simulink model "Kalman_FullSystem"  (R2024a)
settings: Solver=FixedStepAuto  StartTime=0.0  StopTime=0.05  FixedStep=0.05  RelTol=1e-3
model workspace (MAT data in the model file):
  Delta_t = 0.1
  J1 = 0.833333333333
  J2 = 1.08333333333
  J3 = 0.416666666667
  NoiseCov = [0.5  0  0  0  0  0; 0  0.5  0  0  0  0; 0  0  0.5  0  0  0; 0  0  0  0.5  0  0; 0  0  0  0  0.5  0; 0  0  0  0  0  0.5]
  Orbit_Incl = 51.6
  Q_identity = [0.05  0  0  0  0  0  0; 0  0.05  0  0  0  0  0; 0  0  0.05  0  0  0  0; 0  0  0  0.05  0  0  0; 0  0  0  0  0.05  0  0; 0  0  0  0  0  0.05  0; 0  0  0  0  0  0  0.05]
  Sig = Simulink.Signal
  Sig.DataType = 'auto'
  Sig.Dimensions = -1
  Sig.DimensionsMode = 'auto'
  Sig.Complexity = 'auto'
  Sig.SampleTime = -1
  Sig.SamplingMode = 'auto'
  Sig1 = Simulink.Signal
  Sig1.DataType = 'auto'
  Sig1.Dimensions = -1
  Sig1.DimensionsMode = 'auto'
  Sig1.Complexity = 'auto'
  Sig1.SampleTime = -1
  Sig1.SamplingMode = 'auto'
  controlRun = 1
  jd_input = 2458850.00006
  m = 100
  n = 7
  prev_torque_input = [4.02125178476e-05; -0.000240074266532; 0.000969921285444]
  q_ff_in = [0.768162333731 -0.000607721012165 0.00073835510125 -0.64025441392]
  q_mea = [0.201779427007 -0.600440780835 -0.499157225709 -0.59126812494]
  s_input = [0.0589841167561  0.00581351479597  0.00668594935891  -0.00630732370495  0.000663483023899  0.00184880164458  0.000570366934632; 0.00581351479597  0.0937594050574  0.0387635496011  -0.0430050360951  0.000555134956355  0.00180643488778  -0.00190339065861; 0.00668594935891  0.0387635496011  0.103662181174  -0.0426676946457  -0.0011343563344  0.00228890389951  0.000237159003537; -0.00630732370495  -0.0430050360951  -0.0426676946457  0.116378630936  0.0019375862402  -0.00189390453411  0.00103186473468; 0.000663483023899  0.000555134956355  -0.0011343563344  0.0019375862402  0.134971771072  -0.000682723438692  0.000145669100888; 0.00184880164458  0.00180643488778  0.00228890389951  -0.00189390453411  -0.000682723438692  0.134976824741  -0.00135891657435; 0.000570366934632  -0.00190339065861  0.000237159003537  0.00103186473468  0.000145669100888  -0.00135891657435  0.134973743075]
  s_input_cons = [1.94870414  1.25588909  1.4416761  1.0780205  1.49168854  1.53894753  1.37981514; 1.25588909  2.30599344  1.57766712  1.62980068  1.46050557  1.31460547  1.13813509; 1.4416761  1.57766712  1.70958392  1.12140846  1.38322267  1.58836736  1.34392315; 1.0780205  1.62980068  1.12140846  1.77837393  1.21690337  0.94427956  1.46043147; 1.49168854  1.46050557  1.38322267  1.21690337  2.06327445  1.39185931  1.33424815; 1.53894753  1.31460547  1.58836736  0.94427956  1.39185931  2.02772691  1.7277207; 1.37981514  1.13813509  1.34392315  1.46043147  1.33424815  1.7277207  2.16380015]
  savedTorque = [0.000657725470141; -0.000240297847613; -0.000713900658607]
  t_step = 0.05
  v_icrf_input = [-949481.777156 -889776.036157 4371.77407199]
  w_mea = [0.000477892534013 0.0173144207751 0.0745768968359]
  x_icrf_input = [-3388291.56974 3592736.49121 -4663347.3899]
  x_icrf_input_cons = [3649700 3308200 -4676600]
  x_input = [0.411501608148; -0.308732372219; -0.291057996427; -0.806620103613; -0.492262126493; 0.179846356615; 0.534305378558]
  x_input_cons = [0.2; 0.6; 0.5; 0.59160797831; 0.1; 0.4; 0.9]
libraries: aerolibsatdyn x2, aerolibtransform2 x2, aerolibutil x2
settings Model: Creator=alenachan  LastModifiedBy=ruimi

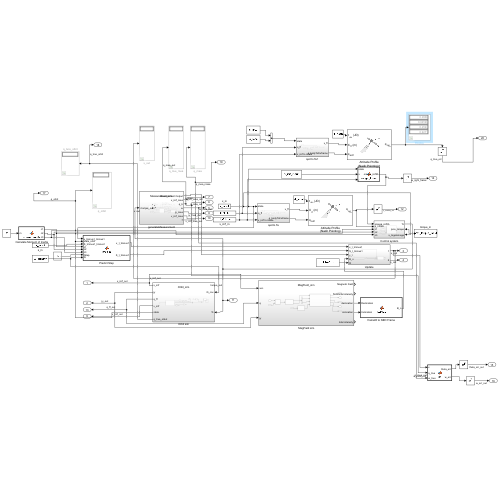
[thumbnail: Simulink's stored preview of the top-level diagram]
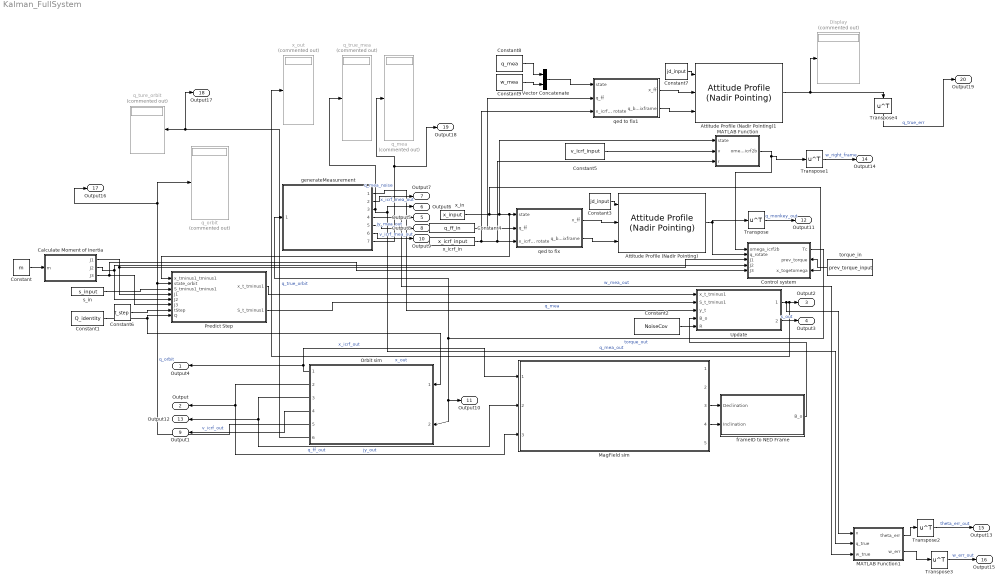
== system Kalman_FullSystem ==
  " Calculate Moment of Inertia" : MATLAB Function  Priority=10  TreatAsAtomicUnit=on
  Attitude Profile (Nadir Pointing) : aerolibsatdyn/Attitude Profile (Nadir Pointing)  Priority=3  outputError=on  outputFinalAttitude=off  portFrame=Fixed-frame  pointingMode=Custom  celestialTarget=Sun  tunablePointing=off  primaryAlignmentSrc=Dialog  primaryAlignment=[0 0 1]  secondaryAlignmentSrc=Dialog  secondaryAlignment=[1 0 0]  constraintFrame=ICRF  primaryConstraintSrc=Dialog  primaryConstraint=[1 0 0]  secondaryConstraintSrc=Dialog  secondaryConstraint=[0 1 0]
  Attitude Profile (Nadir Pointing)1 : aerolibsatdyn/Attitude Profile (Nadir Pointing)  Priority=3  outputError=on  outputFinalAttitude=off  portFrame=Fixed-frame  pointingMode=Custom  celestialTarget=Sun  tunablePointing=off  primaryAlignmentSrc=Dialog  primaryAlignment=[0 0 1]  secondaryAlignmentSrc=Dialog  secondaryAlignment=[1 0 0]  constraintFrame=ICRF  primaryConstraintSrc=Dialog  primaryConstraint=[1 0 0]  secondaryConstraintSrc=Dialog  secondaryConstraint=[0 1 0]
  Constant : Constant  Value=m
  Constant1 : Constant  Value=Q_identity
  Constant2 : Constant  Value=NoiseCov
  Constant3 : Constant  Value=jd_input
  Constant4 : Constant  Value=q_ff_in
  Constant5 : Constant  Value=v_icrf_input
  Constant6 : Constant  Value=t_step
  Constant7 : Constant  Value=jd_input
  Constant8 : Constant  Value=q_mea
  Constant9 : Constant  Value=w_mea
  Control system : Subsystem  Priority=4
      settings: PortSchema="{\"entries\":[{\"content\":{\"sides\":[{\"content\":{\"connectorIds\":[\"In1\",\"In2\",\"In3\",\"In4\",\"In5\"]},\"type\":\"ConnectorPlacement.EquallySpacedRectSide\",\"uuid\":\"8eb5f269-cc65-4267-936a-9f0f4ccd4d18\"},{\"content\":{\"connectorIds\":[\"Out1\",\"In6\",\"In7\"],\"side\":\"RIGHT\"},\"type\":\"ConnectorPlacement.EquallySpacedRectSide\",\"uuid\":\"3df96c14-e4ae-45ba-8fc0-de3a9fdcf55a\"},{\"content\":{\"side\":\"TOP\"},\"type\":\"ConnectorPlacement.EquallySpacedRectSide\",\"uuid\":\"e3effbcc-2fcc-4dea-811c-5aa639521533\"}]},\"type\":\"ConnectorPlacement.EquallySpacedConnector\",\"uuid\":\"93bbc224-b85a-4291-8bf8-2645c40efc9b\"}],\"packageUris\":[\"http://schema.mathworks.com/mf0/Connector/R2020b\"],\"version\":\"1.0\"}"
  Display : Display  Commented=on
  MATLAB Function : MATLAB Function  TreatAsAtomicUnit=on
  MATLAB Function1 : MATLAB Function  TreatAsAtomicUnit=on
  MagField sim : Subsystem  Priority=8  ReferencedSubsystem=MagField_sim
  Orbit sim : Subsystem  Priority=7  ReferencedSubsystem=Orbit_sim
  Predict Step : MATLAB Function  Priority=11  TreatAsAtomicUnit=on
  Transpose{,1..4} (5 alike) : Math  Operator=transpose
  Update : Subsystem  Priority=12
  Vector Concatenate : Concatenate
  frameID to NED Frame : MATLAB Function  Priority=9  TreatAsAtomicUnit=on
  generateMeasurement : Subsystem  Priority=5  ReferencedSubsystem=Measurement_sim
  q_mea : Display  Commented=on
  q_orbit : Display  Commented=on
  q_true_mea : Display  Commented=on
  q_ture_orbit : Display  Commented=on
  qed to fix : Subsystem  Priority=2
  qed to fix1 : Subsystem  Priority=2
  s_in : Constant  Priority=1  Value=s_input
  torque_in : Constant  Value=prev_torque_input
  x_icrf_in : Constant  Value=x_icrf_input
  x_in : Constant  Value=x_input
  x_out : Display  Commented=on
  Output4 : Outport
  Output : Outport  Port=2
  Output2 : Outport  Port=3
  Output3 : Outport  Port=4
  Output5 : Outport  Port=5
  Output6 : Outport  Port=6
  Output7 : Outport  Port=7
  Output8 : Outport  Port=8
  Output1 : Outport  Port=9
  Output9 : Outport  Port=10
  Output10 : Outport  Port=11
  Output11 : Outport  Port=12
  Output12 : Outport  Port=13
  Output14 : Outport  Port=14
  Output13 : Outport  Port=15
  Output15 : Outport  Port=16
  Output16 : Outport  Port=17
  Output17 : Outport  Port=18
  Output18 : Outport  Port=19
  Output19 : Outport  Port=20
  wires:
  Control system/1(Tc) -> Output10/1, Orbit sim/2, generateMeasurement/1  "torque_out"
  MagField sim/3 -> frameID to NED Frame/1(Declination)
  MagField sim/4 -> frameID to NED Frame/2(Inclination)
  frameID to NED Frame/1(B_o) -> Update/4(B_o)
  Orbit sim/2 -> MagField sim/3, Output/1  "jy_out"
  Orbit sim/1 -> MagField sim/1, Output4/1  "x_icrf_out"
  Constant/1 -> " Calculate Moment of Inertia"/1(m)
  " Calculate Moment of Inertia"/1(J1) -> Predict Step/4(J1), Control system/3(J1)
  " Calculate Moment of Inertia"/2(J2) -> Control system/4(J2), Predict Step/5(J2)
  " Calculate Moment of Inertia"/3(J3) -> Predict Step/6(J3), Control system/5(J3)
  Constant1/1 -> Orbit sim/1, Predict Step/8(Q)
  x_in/1 -> Control system/7(x_togetomega), MATLAB Function/1(state), Predict Step/1(x_tminus1_tminus1), qed to fix/1(state)
  s_in/1 -> Predict Step/3(S_tminus1_tminus1)
  x_icrf_in/1 -> qed to fix1/3(x_icrf to rotate), MATLAB Function/3(r), qed to fix/3(x_icrf to rotate)
  Predict Step/1(x_t_tminus1) -> Update/1(x_t_tminus1)
  Predict Step/2(S_t_tminus1) -> Update/2(S_t_tminus1)
  Constant2/1 -> Update/5(R)
  Update/1(1) -> MATLAB Function1/1(x), x_out/1, Output2/1  "x_out"
  Update/2(2) -> Output3/1  "s_out"
  Orbit sim/3 -> MagField sim/2, Output12/1  "q_ff_out"
  generateMeasurement/2 -> Output7/1  "x_icrf_mea_out"
  generateMeasurement/5 -> Output8/1  "jy_mea_out"
  Orbit sim/4 -> Output1/1  "v_icrf_out"
  generateMeasurement/6 -> Output9/1  "v_icrf_mea_out"
  torque_in/1 -> Control system/6(prev_torque)
  Transpose/1 -> Output11/1  "q_monkey_out"
  Constant3/1 -> Attitude Profile (Nadir Pointing)/1
  qed to fix/2(q_bodyToFixframe) -> Attitude Profile (Nadir Pointing)/3
  Constant4/1 -> qed to fix1/2(q_ff), qed to fix/2(q_ff)
  qed to fix/1(x_ff) -> Attitude Profile (Nadir Pointing)/2
  Constant6/1 -> Predict Step/7(tStep)
  Orbit sim/5 -> Output16/1, q_orbit/1, Predict Step/2(state_orbit)  "q_orbit"
  Attitude Profile (Nadir Pointing)/1 -> Transpose/1, Control system/2(q_rotate)
  Constant5/1 -> MATLAB Function/2(v)
  MATLAB Function/1(omega_icrf2b) -> Transpose1/1, Control system/1(omega_icrf2b)
  Transpose1/1 -> Output14/1  "w_right_frame"
  Transpose2/1 -> Output13/1  "theta_err_out"
  MATLAB Function1/2(w_err) -> Transpose3/1
  Transpose3/1 -> Output15/1  "w_err_out"
  generateMeasurement/4 -> MATLAB Function1/3(w_true), Output5/1  "w_mea_out"
  generateMeasurement/3 -> Output6/1, MATLAB Function1/2(q_true), q_true_mea/1  "q_mea_out"
  MATLAB Function1/1(theta_err) -> Transpose2/1
  Orbit sim/6 -> Output17/1, q_ture_orbit/1  "q_true_orbit"
  generateMeasurement/1 -> Update/3(y_t)  "q_mea"
  generateMeasurement/7 -> Output18/1, q_mea/1  "q_mea_noise"
  Constant7/1 -> Attitude Profile (Nadir Pointing)1/1
  qed to fix1/1(x_ff) -> Attitude Profile (Nadir Pointing)1/2
  qed to fix1/2(q_bodyToFixframe) -> Attitude Profile (Nadir Pointing)1/3
  Constant8/1 -> Vector Concatenate/1
  Constant9/1 -> Vector Concatenate/2
  Vector Concatenate/1 -> qed to fix1/1(state)
  Attitude Profile (Nadir Pointing)1/1 -> Display/1, Transpose4/1
  Transpose4/1 -> Output19/1  "q_true_err"

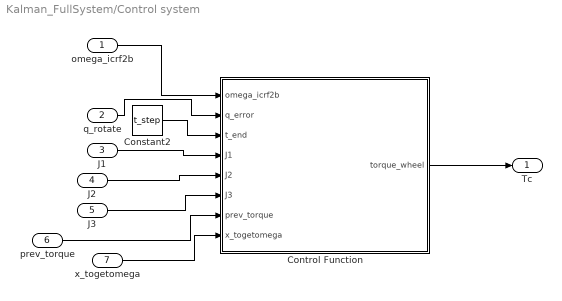
== system Kalman_FullSystem/Control system ==
  omega_icrf2b : Inport
  q_rotate : Inport  Port=2
  J1 : Inport  Port=3
  J2 : Inport  Port=4
  J3 : Inport  Port=5
  prev_torque : Inport  Port=6
  x_togetomega : Inport  Port=7
  Constant2 : Constant  Value=t_step
  Control Function : MATLAB Function  TreatAsAtomicUnit=on
  Tc : Outport
  wires:
  Constant2/1 -> Control Function/3(t_end)
  Control Function/1(torque_wheel) -> Tc/1
  q_rotate/1 -> Control Function/2(q_error)
  J1/1 -> Control Function/4(J1)
  J2/1 -> Control Function/5(J2)
  J3/1 -> Control Function/6(J3)
  prev_torque/1 -> Control Function/7(prev_torque)
  x_togetomega/1 -> Control Function/8(x_togetomega)
  omega_icrf2b/1 -> Control Function/1(omega_icrf2b)

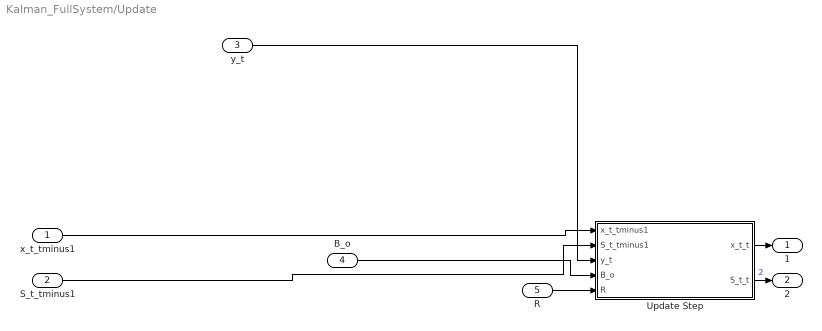
== system Kalman_FullSystem/Update ==
  x_t_tminus1 : Inport
  S_t_tminus1 : Inport  Port=2
  y_t : Inport  Port=3
  B_o : Inport  Port=4
  R : Inport  Port=5
  Update Step : MATLAB Function  TreatAsAtomicUnit=on
  1 : Outport
  2 : Outport  Port=2
  wires:
  y_t/1 -> Update Step/3(y_t)
  Update Step/2(S_t_t) -> 2/1  "2"
  B_o/1 -> Update Step/4(B_o)
  S_t_tminus1/1 -> Update Step/2(S_t_tminus1)
  x_t_tminus1/1 -> Update Step/1(x_t_tminus1)
  R/1 -> Update Step/5(R)
  Update Step/1(x_t_t) -> 1/1

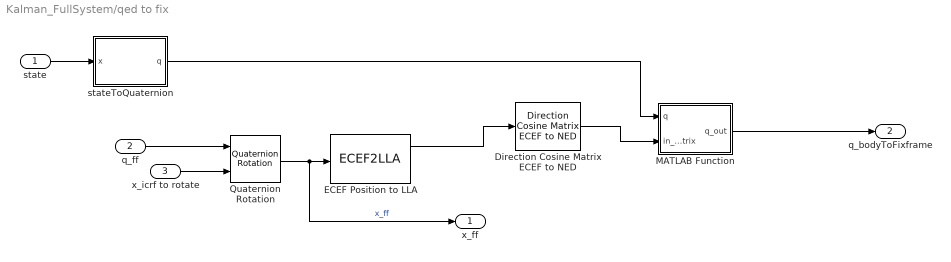
== system Kalman_FullSystem/qed to fix ==
  state : Inport
  q_ff : Inport  Port=2
  x_icrf to rotate : Inport  Port=3
  Direction Cosine Matrix ECEF to NED : aerolibtransform2/Direction Cosine Matrix ECEF to NED
  ECEF Position to LLA : ECEF2LLA
  MATLAB Function : MATLAB Function  TreatAsAtomicUnit=on
  Quaternion Rotation : aerolibutil/Quaternion Rotation
  stateToQuaternion : MATLAB Function  TreatAsAtomicUnit=on
  x_ff : Outport
  q_bodyToFixframe : Outport  Port=2
  wires:
  state/1 -> stateToQuaternion/1(x)
  Quaternion Rotation/1 -> x_ff/1, ECEF Position to LLA/1  "x_ff"
  x_icrf to rotate/1 -> Quaternion Rotation/2
  ECEF Position to LLA/1 -> Direction Cosine Matrix ECEF to NED/1
  Direction Cosine Matrix ECEF to NED/1 -> MATLAB Function/2(in_matrix)
  stateToQuaternion/1(q) -> MATLAB Function/1(q)
  MATLAB Function/1(q_out) -> q_bodyToFixframe/1
  q_ff/1 -> Quaternion Rotation/1

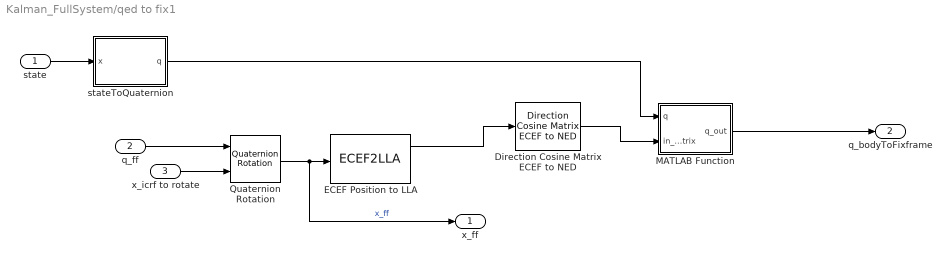
== system Kalman_FullSystem/qed to fix1 ==
  state : Inport
  q_ff : Inport  Port=2
  x_icrf to rotate : Inport  Port=3
  Direction Cosine Matrix ECEF to NED : aerolibtransform2/Direction Cosine Matrix ECEF to NED
  ECEF Position to LLA : ECEF2LLA
  MATLAB Function : MATLAB Function  TreatAsAtomicUnit=on
  Quaternion Rotation : aerolibutil/Quaternion Rotation
  stateToQuaternion : MATLAB Function  TreatAsAtomicUnit=on
  x_ff : Outport
  q_bodyToFixframe : Outport  Port=2
  wires:
  state/1 -> stateToQuaternion/1(x)
  Quaternion Rotation/1 -> x_ff/1, ECEF Position to LLA/1  "x_ff"
  x_icrf to rotate/1 -> Quaternion Rotation/2
  ECEF Position to LLA/1 -> Direction Cosine Matrix ECEF to NED/1
  Direction Cosine Matrix ECEF to NED/1 -> MATLAB Function/2(in_matrix)
  stateToQuaternion/1(q) -> MATLAB Function/1(q)
  MATLAB Function/1(q_out) -> q_bodyToFixframe/1
  q_ff/1 -> Quaternion Rotation/1

== matlab function Kalman_FullSystem/Control system/Control Function ==
  data: omega_icrf2b input; q_error input; t_end input; torque_wheel output size=[3 1]; J1 input; J2 input; J3 input; prev_torque input; x_togetomega input
function torque_wheel = fcn(omega_icrf2b, q_error, t_end, J1, J2, J3, prev_torque, x_togetomega)
coder.extrinsic("get_param");
coder.extrinsic("getVariable");
coder.extrinsic("quat2angle");

mdlWks = get_param('Kalman_FullSystem','ModelWorkspace');
ctrlRn = getVariable(mdlWks,'controlRun');
if ~ctrlRn
    %disp('enter Control');

    if(norm(x_togetomega(5:7)) > 0.15)
        torque_wheel_calc = -0.8*x_togetomega(5:7);
    else
        theta = (2*acos(q_error(1))); % magnitude
        if (theta>pi)
            theta=2* pi-theta;
        end
        direction = [q_error(2);q_error(3); q_error(4)]/(sin(theta/2)); %3d-vector
        omega_cur_indir=dot(omega_icrf2b*t_end,direction);
        acc = ((theta - omega_cur_indir*t_end)* 2)/(t_end^2); % magnitude
        acc_directed = acc*direction; %3d-vector
        
        I_sate = [J1,0,0; 0,J2,0; 0,0,J3]; % define moment of inertia (same for every wheel)
        torque_wheel_calc = 0.9*I_sate * acc_directed + 0.1*prev_torque; % 3-d vector; 0.1 is momentum coefficient
    end

    max_torque = .001; % 0.824 * 10^(-2); %reasonable estimate from CSI document
    if norm(torque_wheel_calc) > max_torque % scale to maximum allowed magnitude
        % disp("Torque is beyond physical limit.");
        torque_wheel = (max_torque/norm(torque_wheel_calc))* torque_wheel_calc;
    else
        torque_wheel = torque_wheel_calc;
    end

    assignin(mdlWks,'savedTorque', torque_wheel);
    assignin(mdlWks,'controlRun', true);    
else
    %disp('skipped control');
    torque_wheel = getVariable(mdlWks,'savedTorque'); % this ensures that value doesn't zero out after multiple runs
end

== matlab function Kalman_FullSystem/qed to fix1/MATLAB Function ==
  data: q input; in_matrix input; q_out output
function q_out= fcn(q, in_matrix)
inv_m = inv(in_matrix);
q_second = rotm2quat(inv_m);
q_first = quatconj(q);
q_out = transpose(quatmultiply(q_second,q_first));

== matlab function Kalman_FullSystem/qed to fix1/stateToQuaternion ==
  data: x input; q output
function q = getq(x)
q_temp = x(1:4);
q = transpose(q_temp);
end

== matlab function Kalman_FullSystem/Update/Update Step ==
  data: x_t_tminus1 input; x_t_t output; S_t_tminus1 input; y_t input; S_t_t output; B_o input; R input
function [x_t_t, S_t_t] = update(x_t_tminus1, S_t_tminus1, y_t, B_o, R)

H_out = H(x_t_tminus1, B_o);
x_t_t = zeros(7,1);
%Kalman Gain
%temp=(H_out*S_t_tminus1*transpose(H_out) + R);
K = S_t_tminus1 * transpose(H_out)/(H_out*S_t_tminus1*transpose(H_out) + R);
%disp('update');
%Update
% temp5=y_t - h_t(x_t_tminus1, B_o);
% temp2=norm(y_t - h_t(x_t_tminus1, B_o));
% temp4= K * (y_t - h_t(x_t_tminus1, B_o));
% temp3=norm(K * (y_t - h_t(x_t_tminus1, B_o)));

%additive
x_t_t = x_t_tminus1 + K * (y_t - h_t(x_t_tminus1, B_o));
x_t_t(1:4)=x_t_t(1:4)/norm(x_t_t(1:4));


% %multiplicative
% x_t_t_add = x_t_tminus1 + K * (y_t - h_t(x_t_tminus1, B_o));
% x_t_t(5:7) = x_t_t_add(5:7);
% del_x =  (K * (y_t - h_t(x_t_tminus1, B_o))); 
% del_q = del_x(1:4)/norm(del_x(1:4));
% x_t_t_mul = transpose(quatmultiply(transpose(x_t_tminus1(1:4)),transpose(del_q)));
% x_t_t(1:4) = x_t_t_mul;


S_t_t = (eye(7) - K*H_out)*S_t_tminus1;

end

== matlab function Kalman_FullSystem/Predict Step ==
  data: x_tminus1_tminus1 input; state_orbit input; x_t_tminus1 output; S_tminus1_tminus1 input; S_t_tminus1 output; J1 input; J2 input; J3 input; tStep input; Q input
function [x_t_tminus1, S_t_tminus1]= predict(x_tminus1_tminus1,state_orbit, S_tminus1_tminus1, J1,J2,J3, tStep, Q)


x_t_tminus1 = state_orbit; %use state from orbit with noise
% x_t_tminus1 = feval(f_t,x_tminus1_tminus1);
F_tminus1 = F(x_tminus1_tminus1, J1,J2,J3,tStep);
%disp('predict');
S_t_tminus1 = F_tminus1 * S_tminus1_tminus1 * transpose(F_tminus1) +Q;

== matlab function Kalman_FullSystem/qed to fix/MATLAB Function ==
  data: q input; in_matrix input; q_out output
function q_out= fcn(q, in_matrix)
inv_m = inv(in_matrix);
q_second = rotm2quat(inv_m);
q_first = quatconj(q);
q_out = transpose(quatmultiply(q_second,q_first));

== matlab function Kalman_FullSystem/qed to fix/stateToQuaternion ==
  data: x input; q output
function q = getq(x)
q_temp = x(1:4);
q = transpose(q_temp);
end

== matlab function Kalman_FullSystem/frameID to NED Frame ==
  data: Declination input; Inclination input; B_o output
function B_o= ID2NED(Declination,Inclination)

[Down_dir,Omega_dir,Other_dir] = MagID2NED(Inclination,Declination);
B_o = [Down_dir;Omega_dir;Other_dir]/norm([Down_dir,Omega_dir,Other_dir]);
%disp('enter NED')

end

== matlab function Kalman_FullSystem/MATLAB Function ==
  data: state input; v input; omega_icrf2b output; r input
function omega_icrf2b = omega_frame(state,v,r)
omega_ned2b = state(5:7);
omega_icrf2ned = -cross(r,v)/norm(r)^2;
omega_icrf2b = omega_ned2b + omega_icrf2ned;

== matlab function Kalman_FullSystem/MATLAB Function1 ==
  data: x input; theta_err output; q_true input; w_true input; w_err output
function [theta_err, w_err]= fcn(x, q_true, w_true)
theta_est = 2*acos(x(1));
theta_true = 2*acos(q_true(1));
theta_err = theta_est - theta_true;
w_err = transpose(x(5:7))-w_true;

== matlab function Kalman_FullSystem/ Calculate Moment of Inertia ==
  data: m input; J1 output; J2 output; J3 output
function [J1,J2,J3]=momentInertia(m)
J1 = m/120;
J2 = 13*m/1200;
J3 = 5*m/1200;
coder.extrinsic("get_param");
mdlWks = get_param('Kalman_FullSystem','ModelWorkspace');
assignin(mdlWks,"J1",J1)
assignin(mdlWks,"J2",J2)
assignin(mdlWks,"J3",J3)
end
